simulink model "MoPhongLaySoLieu"  (R2018a)
settings: Solver=FixedStepAuto  StartTime=0.0  StopTime=30  FixedStep=0.01  RelTol=1e-3
values from neighbouring files (symbols this model uses):
  l = 0.5    [ThongSo.m]
  M = 1    [ThongSo.m]
  m = 0.1    [ThongSo.m]
settings Model: Creator=vanph  LastModifiedBy=vutie
settings DataIOCC: ReturnWorkspaceOutputs=on
settings DebuggingCC: UnconnectedInputMsg=none  UnconnectedOutputMsg=none  UnconnectedLineMsg=none  SFMachineParentedDataDiag=error
settings ModelReferenceCC: EnableRefExpFcnMdlSchedulingChecks=off
settings SFSimCC: SimUseLocalCustomCode=on
settings RTWCC: Description=Generic Real-Time Target  RTWUseLocalCustomCode=on

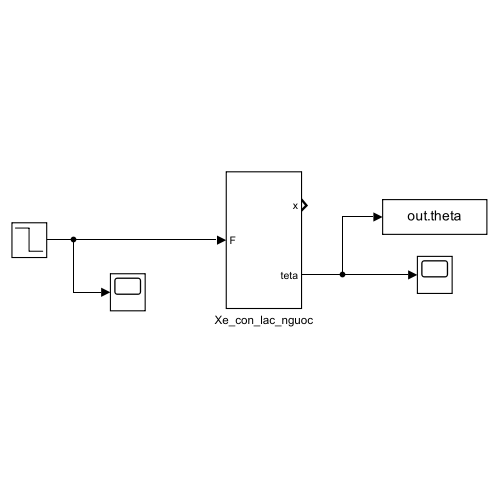
[thumbnail: Simulink's stored preview of the top-level diagram]
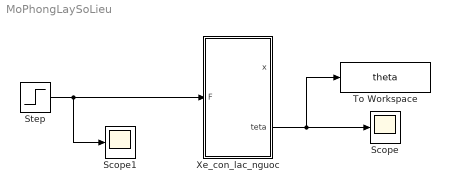
== system MoPhongLaySoLieu ==
  Scope : Scope
  Scope1 : Scope
  Step : Step  Time=5  Before=1  After=0  SampleTime=0
  To Workspace : ToWorkspace  VariableName=theta  SaveFormat=Timeseries  SampleTime=-1
  Xe_con_lac_nguoc : Subsystem
  wires:
  Xe_con_lac_nguoc/2(teta) -> To Workspace/1, Scope/1
  Step/1 -> Xe_con_lac_nguoc/1(F), Scope1/1

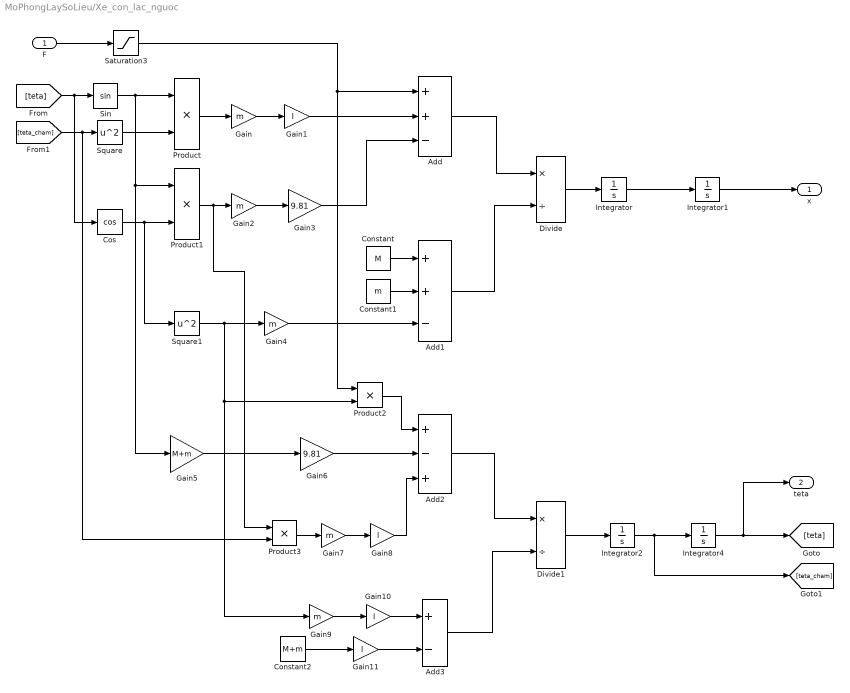
== system MoPhongLaySoLieu/Xe_con_lac_nguoc ==
  F : Inport
  Add : Sum  Inputs=++-
  Add1 : Sum  Inputs=++-
  Add2 : Sum  Inputs=+-+
  Add3 : Sum  Inputs=+-
  Constant : Constant  Value=M
  Constant1 : Constant  Value=m
  Constant2 : Constant  Value=M+m
  Cos : Trigonometry  Operator=cos
  Divide : Product  Inputs=*/
  Divide1 : Product  Inputs=*/
  Gain{,2,4,7,9} (5 alike) : Gain  Gain=m
  Gain{1,8,10..11} (4 alike) : Gain  Gain=l
  Gain3 : Gain  Gain=9.81
  Gain5 : Gain  Gain=M+m
  Gain6 : Gain  Gain=9.81
  Integrator{,1..2,4} (4 alike) : Integrator
  Product{,1..3} (4 alike) : Product
  Saturation3 : Saturate  UpperLimit=40  LowerLimit=-40
  Sin : Trigonometry
  Square : Math  Operator=square  SaturateOnIntegerOverflow=on
  Square1 : Math  Operator=square  SaturateOnIntegerOverflow=on
  x : Outport
  teta : Outport  Port=2
  wires:
  Add1/1 -> Divide/2
  Product3/1 -> Gain7/1
  Gain3/1 -> Add/3
  Gain6/1 -> Add2/2
  Cos/1 -> Square1/1, Product1/2
  Gain4/1 -> Add1/3
  Add2/1 -> Divide1/1
  [teta_cham] -> Product3/2, Square/1
  Gain7/1 -> Gain8/1
  Product1/1 -> Product3/1, Gain2/1
  Constant/1 -> Add1/1
  Gain10/1 -> Add3/1
  Constant2/1 -> Gain11/1
  [teta] -> Cos/1, Sin/1
  Sin/1 -> Gain5/1, Product1/1, Product/1
  Integrator/1 -> Integrator1/1
  Gain/1 -> Gain1/1
  Product2/1 -> Add2/1
  Add3/1 -> Divide1/2
  Integrator4/1 -> [teta], teta/1
  Gain8/1 -> Add2/3
  Gain2/1 -> Gain3/1
  Square1/1 -> Gain9/1, Product2/2, Gain4/1
  Gain9/1 -> Gain10/1
  Square/1 -> Product/2
  Saturation3/1 -> Add/1, Product2/1
  Product/1 -> Gain/1
  Gain5/1 -> Gain6/1
  Gain1/1 -> Add/2
  Divide/1 -> Integrator/1
  F/1 -> Saturation3/1
  Integrator1/1 -> x/1
  Gain11/1 -> Add3/2
  Constant1/1 -> Add1/2
  Add/1 -> Divide/1
  Divide1/1 -> Integrator2/1
  Integrator2/1 -> Integrator4/1, [teta_cham]
